simulink model "untitled"  (Simulink 9.2)
settings: Solver=ode45  StartTime=0.0  StopTime=10  FixedStep=100000  RelTol=1e-3  EnableMultiTasking=on
settings Model: Creator=student  LastModifiedBy=murad
settings OptimizationCC: ExpressionDepthLimit=2147483647
settings DebuggingCC: SolverPrmCheckMsg=warning

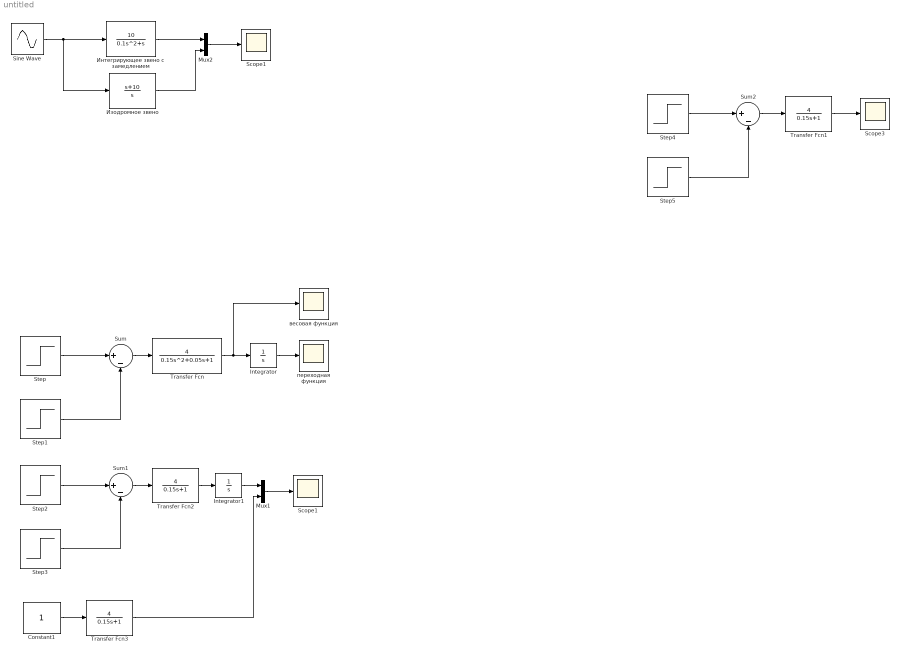
== system untitled ==
  Constant1 : Constant
  Integrator : Integrator
  "Integrator1 " : Integrator
  Mux1 : Mux  Inputs=2
  Mux2 : Mux  Inputs=2
  Scope1 : Scope
  "Scope1 " : Scope
  Scope3 : Scope
  Sine Wave : Sin  Frequency=15  SampleTime=0
  Step : Step  Time=0  SampleTime=0
  Step1 : Step  Time=0.001  SampleTime=0
  Step2 : Step  Time=0  After=2  SampleTime=0
  Step3 : Step  Time=0.5  After=2  SampleTime=0
  "Step4 " : Step  Time=0  After=100  SampleTime=0
  "Step5 " : Step  Time=0.01  After=100  SampleTime=0
  Sum : Sum  Inputs=|+-
  Sum1 : Sum  Inputs=|+-
  Sum2 : Sum  Inputs=|+-
  Transfer Fcn : TransferFcn  Numerator=[4]  Denominator=[0.15 0.05 1]
  "Transfer Fcn1 " : TransferFcn  Numerator=[4]  Denominator="[0.15  1]"
  "Transfer Fcn2 " : TransferFcn  Numerator=[4]  Denominator=[0.15 1]
  Transfer Fcn3 : TransferFcn  Numerator=[4]  Denominator=[0.15 1]
  Изодромное звено : TransferFcn  Numerator=[1 10]  Denominator=[1 0]
  Интегрирующее звено с замедлением : TransferFcn  Numerator=[10]  Denominator=[0.1 1 0]
  весовая функция : Scope
  переходная функция : Scope
  wires:
  Step/1 -> Sum/1
  Sum/1 -> Transfer Fcn/1
  Transfer Fcn/1 -> весовая функция/1, Integrator/1
  Step2/1 -> Sum1/1
  Step3/1 -> Sum1/2
  Sum1/1 -> "Transfer Fcn2 "/1
  Constant1/1 -> Transfer Fcn3/1
  Mux1/1 -> "Scope1 "/1
  "Transfer Fcn2 "/1 -> "Integrator1 "/1
  "Integrator1 "/1 -> Mux1/1
  Transfer Fcn3/1 -> Mux1/2
  Integrator/1 -> переходная функция/1
  Step1/1 -> Sum/2
  Интегрирующее звено с замедлением/1 -> Mux2/1
  Mux2/1 -> Scope1/1
  Изодромное звено/1 -> Mux2/2
  "Step4 "/1 -> Sum2/1
  "Step5 "/1 -> Sum2/2
  Sum2/1 -> "Transfer Fcn1 "/1
  "Transfer Fcn1 "/1 -> Scope3/1
  Sine Wave/1 -> Изодромное звено/1, Интегрирующее звено с замедлением/1
